simulink model "OverheadCrane"  (R2014a)
settings: Solver=ode3  StartTime=0.0  StopTime=10.0  FixedStep=0.5  RelTol=1e-3
settings Model: Creator=tri  LastModifiedBy=tri

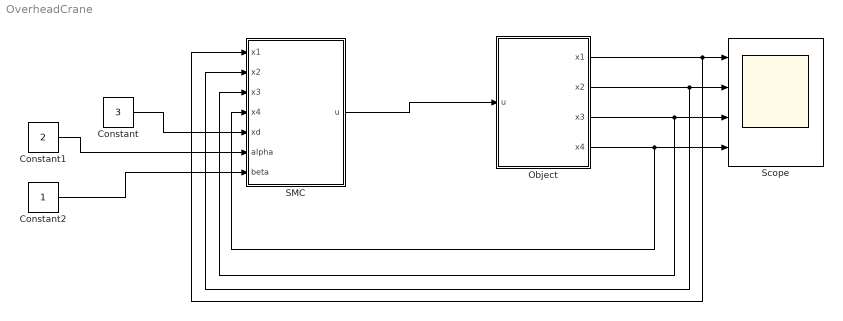
== system OverheadCrane ==
  Constant : Constant  Value=3
  Constant1 : Constant  Value=2
  Constant2 : Constant
  Object : Subsystem
  SMC : Subsystem
  Scope : Scope  NumInputPorts=4
      settings: YMin=-5~-5~-5~-5  YMax=5~5~5~5
  wires:
  Object/1(x1) -> SMC/1(x1), Scope/1
  Object/2(x2) -> SMC/2(x2), Scope/2
  Object/3(x3) -> SMC/3(x3), Scope/3
  SMC/1(u) -> Object/1(u)
  Constant/1 -> SMC/5(xd)
  Object/4(x4) -> SMC/4(x4), Scope/4
  Constant1/1 -> SMC/6(alpha)
  Constant2/1 -> SMC/7(beta)

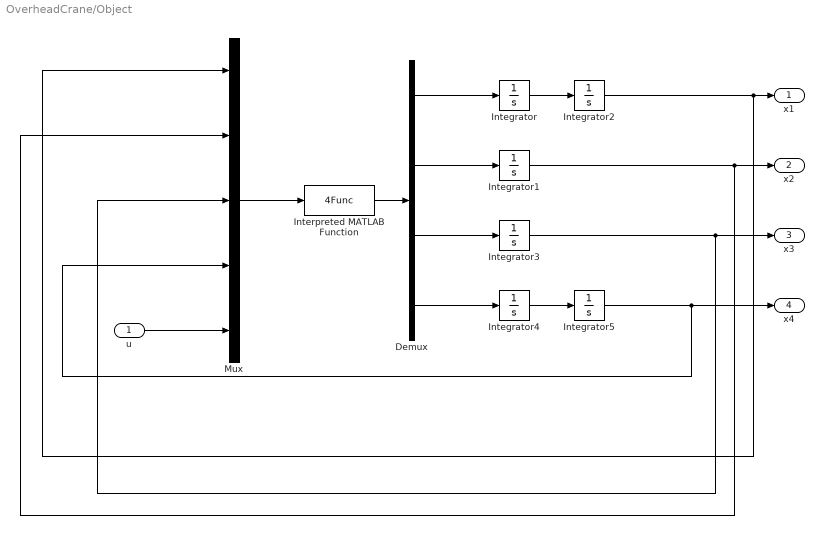
== system OverheadCrane/Object ==
  u : Inport
  Demux : Demux
  Integrator{,1..5} (6 alike) : Integrator
  Interpreted MATLAB Function : MATLABFcn  MATLABFcn=4Func  OutputDimensions=4
  Mux : Mux  Inputs=5
  x1 : Outport
  x2 : Outport  Port=2
  x3 : Outport  Port=3
  x4 : Outport  Port=4
  wires:
  Mux/1 -> Interpreted MATLAB Function/1
  Interpreted MATLAB Function/1 -> Demux/1
  Demux/1 -> Integrator/1
  Demux/3 -> Integrator3/1
  Demux/4 -> Integrator4/1
  Demux/2 -> Integrator1/1
  u/1 -> Mux/5
  Integrator1/1 -> Mux/2, x2/1
  Integrator/1 -> Integrator2/1
  Integrator2/1 -> Mux/1, x1/1
  Integrator3/1 -> Mux/3, x3/1
  Integrator4/1 -> Integrator5/1
  Integrator5/1 -> Mux/4, x4/1

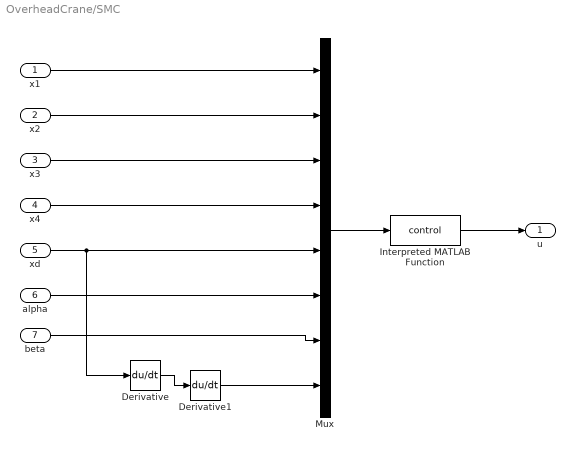
== system OverheadCrane/SMC ==
  x1 : Inport
  x2 : Inport  Port=2
  x3 : Inport  Port=3
  x4 : Inport  Port=4
  xd : Inport  Port=5
  alpha : Inport  Port=6
  beta : Inport  Port=7
  Derivative : Derivative
  Derivative1 : Derivative
  Interpreted MATLAB Function : MATLABFcn  MATLABFcn=control  OutputDimensions=2  SampleTime=1
  Mux : Mux  Inputs=8
  u : Outport
  wires:
  x1/1 -> Mux/1
  x2/1 -> Mux/2
  x3/1 -> Mux/3
  x4/1 -> Mux/4
  xd/1 -> Derivative/1, Mux/5
  alpha/1 -> Mux/6
  beta/1 -> Mux/7
  Mux/1 -> Interpreted MATLAB Function/1
  Interpreted MATLAB Function/1 -> u/1
  Derivative/1 -> Derivative1/1
  Derivative1/1 -> Mux/8
